simulink model "Lab5_EX2"  (R2015a)
settings: Solver=ode45  StartTime=0.0  StopTime=200  RelTol=1e-3
values from neighbouring files (symbols this model uses):
  C = 10*C/100    [RLC.m]    (also in RLC_COMPLEX.m = 10)
  L = 1*L/100    [RLC.m]
  R = 10*R/100    [RLC.m]
settings Model: Creator=Bilal  LastModifiedBy=Bilal

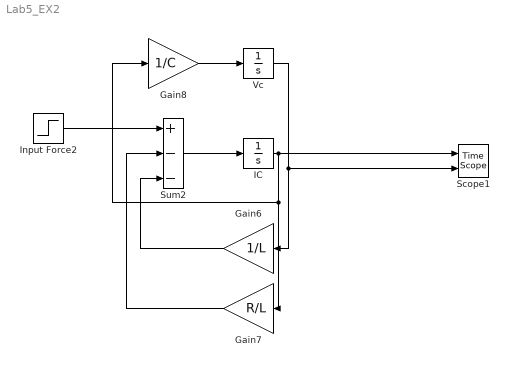
== system Lab5_EX2 ==
  Gain6 : Gain  Gain=1/L
  Gain7 : Gain  Gain=R/L
  Gain8 : Gain  Gain=1/C
  "IC " : Integrator
  Input Force2 : Step  Time=0  After=E/L  SampleTime=0
  Scope1 : TimeScope  NumInputPorts=2
  Sum2 : Sum  Inputs=+--
  "Vc " : Integrator
  wires:
  Sum2/1 -> "IC "/1
  Gain6/1 -> Sum2/3
  "Vc "/1 -> Scope1/2, Gain6/1
  "IC "/1 -> Gain8/1, Gain7/1, Scope1/1
  Gain7/1 -> Sum2/2
  Input Force2/1 -> Sum2/1
  Gain8/1 -> "Vc "/1
